simulink model "wmm_edca_nv1640"  (R2024b)
settings: Solver=VariableStepAuto  StartTime=0.0  StopTime=30  RelTol=1e-3
values from neighbouring files (symbols this model uses):
  m = comm.OFDMModulator('FFTLength',128,'NumGuardBandCarriers',[6;5])    [prueba_wlan.m]
  n = min(n, listos)    [ver_wmm_paquetes.m]
settings Model: Creator=AdrianLopez  LastModifiedBy=AdrianLopez

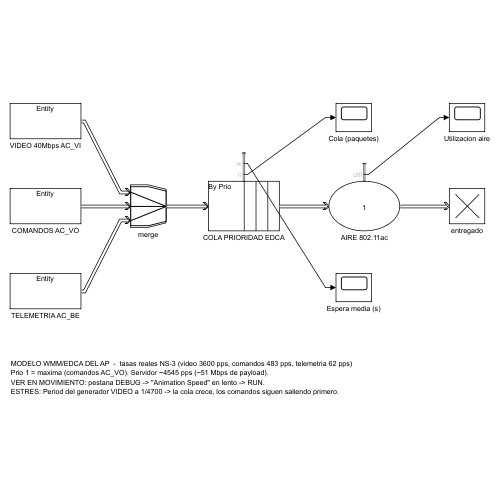
[thumbnail: Simulink's stored preview of the top-level diagram]
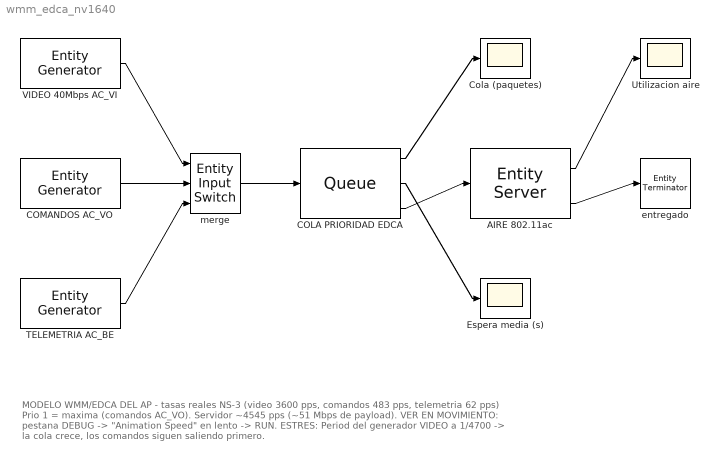
== system wmm_edca_nv1640 ==
  note: MODELO WMM/EDCA DEL AP  -  tasas reales NS-3 (video 3600 pps, comandos 483 pps, telemetria 62 pps)
      | Prio 1 = maxima (comandos AC_VO). Servidor ~4545 pps (~51 Mbps de payload).
      | VER EN MOVIMIENTO: pestana DEBUG -> "Animation Speed" en lento -> RUN.
      | ESTRES: Period del generador VIDEO a 1/4700 -> la cola crece, los comandos siguen saliendo primero.
  AIRE 802.11ac : EntityServer  InputPortMessageModes=m  OutputPortMessageModes=n,m  Capacity=1  ServiceTimeValue=2.2e-4  Utilization=on
      settings: OutputPortMap=o5,o9
  COLA PRIORIDAD EDCA : Queue  InputPortMessageModes=m  OutputPortMessageModes=n,n,m  Capacity=5000  QueueType=Priority  PrioritySource=Prio  NumberEntitiesInBlock=on  AverageWait=on
      settings: OutputPortMap=o1,o2,o5
  COMANDOS AC_VO : EntityGenerator  OutputPortMessageModes=m  Period=1/483  AttributeName=Prio  EntityType=Structured  EntityTypeName=Entity
  Cola (paquetes) : Scope
  Espera media (s) : Scope
  TELEMETRIA AC_BE : EntityGenerator  OutputPortMessageModes=m  Period=1/62  AttributeName=Prio  AttributeInitialValue=3  EntityType=Structured  EntityTypeName=Entity
  Utilizacion aire : Scope
  VIDEO 40Mbps AC_VI : EntityGenerator  OutputPortMessageModes=m  Period=1/3600  AttributeName=Prio  AttributeInitialValue=2  EntityType=Structured  EntityTypeName=Entity
  entregado : EntityTerminator  InputPortMessageModes=m
  merge : EntityInputSwitch  InputPortMessageModes=m,m,m  OutputPortMessageModes=m  NumberInputPorts=3
      settings: InputPortMap=u1,u2,u3
  wires:
  VIDEO 40Mbps AC_VI/1 -> merge/1
  COMANDOS AC_VO/1 -> merge/2
  TELEMETRIA AC_BE/1 -> merge/3
  merge/1 -> COLA PRIORIDAD EDCA/1
  COLA PRIORIDAD EDCA/3 -> AIRE 802.11ac/1
  AIRE 802.11ac/2 -> entregado/1
  COLA PRIORIDAD EDCA/1 -> Cola (paquetes)/1
  COLA PRIORIDAD EDCA/2 -> Espera media (s)/1
  AIRE 802.11ac/1 -> Utilizacion aire/1
